simulink model "Practica_3_simulin_Simscape"  (R2022b)
settings: Solver=VariableStepAuto  StartTime=0.0  StopTime=10  FixedStep=0.001  MaxStep=0.00001  RelTol=1e-3
values from neighbouring files (symbols this model uses):
  b1 = 1000    [DobleP1.m]
  k1 = 16182    [DobleP1.m]
  k2 = 19000    [DobleP1.m]
  m1 = 290    [DobleP1.m]
  m2 = 59    [DobleP1.m]
libraries: fl_lib x11, nesl_utility x4
settings Model: Creator=mluser  LastModifiedBy=mluser

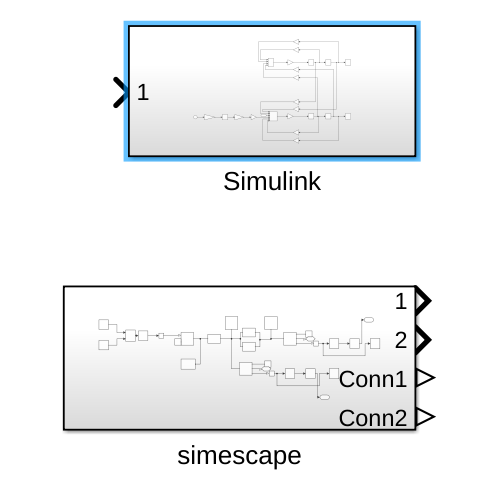
[thumbnail: Simulink's stored preview of the top-level diagram]
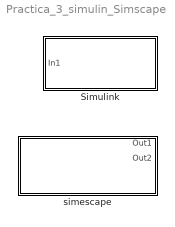
== system Practica_3_simulin_Simscape ==
  Simulink : Subsystem
  simescape : Subsystem

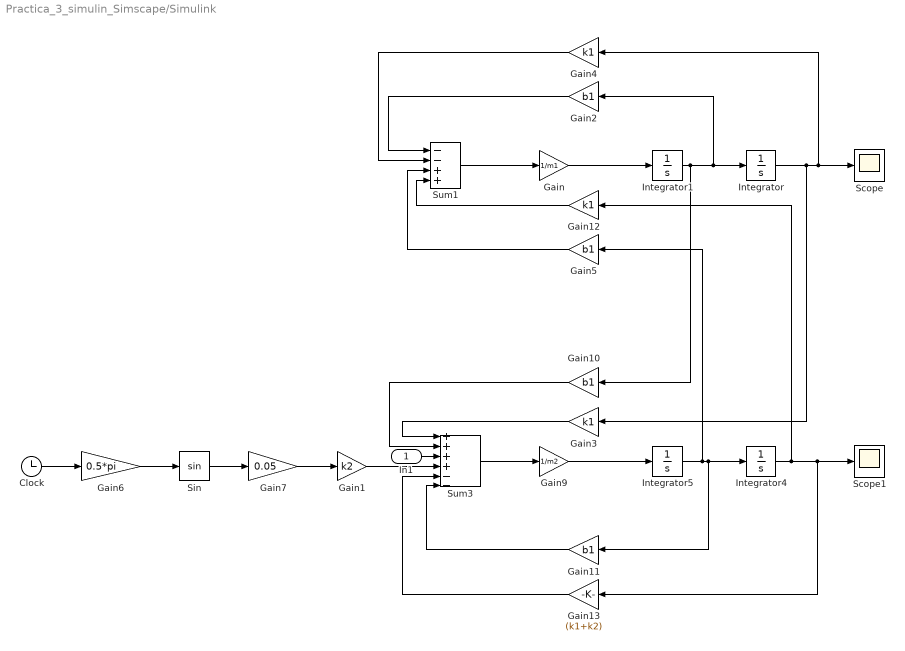
== system Practica_3_simulin_Simscape/Simulink ==
  In1 : Inport
  Clock : Clock
  Gain : Gain  Gain=1/m1
  Gain1 : Gain  Gain=k2
  Gain{2,5,10..11} (4 alike) : Gain  Gain=b1
  Gain12 : Gain  Gain=k1
  Gain13 : Gain  Gain=(k1+k2)
  Gain3 : Gain  Gain=k1
  Gain4 : Gain  Gain=k1
  Gain6 : Gain  Gain=0.5*pi
  Gain7 : Gain  Gain=0.05
  Gain9 : Gain  Gain=1/m2
  Integrator{,1,4..5} (4 alike) : Integrator
  Scope : Scope
  Scope1 : Scope
  Sin : Trigonometry
  Sum1 : Sum  Inputs=--++
  Sum3 : Sum  Inputs=++++--
  wires:
  Clock/1 -> Gain6/1
  Gain2/1 -> Sum1/1
  Sin/1 -> Gain7/1
  Gain9/1 -> Integrator5/1
  Gain10/1 -> Sum3/2
  Sum3/1 -> Gain9/1
  Gain/1 -> Integrator1/1
  Integrator/1 -> Gain4/1, Scope/1, Gain3/1
  Gain3/1 -> Sum3/1
  Gain5/1 -> Sum1/3
  Integrator4/1 -> Gain13/1, Scope1/1, Gain12/1
  Integrator5/1 -> Gain5/1, Gain11/1, Integrator4/1
  Gain11/1 -> Sum3/6
  Gain13/1 -> Sum3/5
  Gain1/1 -> Sum3/4
  Sum1/1 -> Gain/1
  Gain12/1 -> Sum1/4
  In1/1 -> Sum3/3
  Gain6/1 -> Sin/1
  Gain7/1 -> Gain1/1
  Integrator1/1 -> Gain2/1, Integrator/1, Gain10/1
  Gain4/1 -> Sum1/2

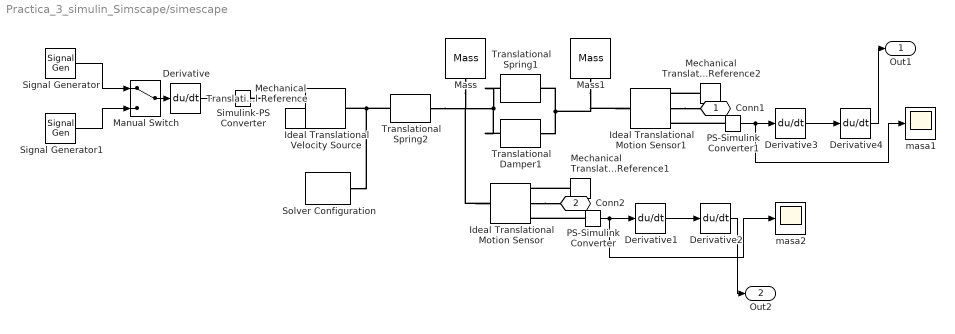
== system Practica_3_simulin_Simscape/simescape ==
  Derivative{,1..4} (5 alike) : Derivative
  Ideal Translational Motion Sensor : fl_lib/Mechanical/Mechanical Sensors/Ideal Translational Motion Sensor  reference=foundation.enum.MeasurementReference.difference  acceleration_port=false  velocity_port=true  position_port=true  offset=0 m
  Ideal Translational Motion Sensor1 : fl_lib/Mechanical/Mechanical Sensors/Ideal Translational Motion Sensor  reference=foundation.enum.MeasurementReference.difference  acceleration_port=false  velocity_port=true  position_port=true  offset=0 m
  Ideal Translational Velocity Source : fl_lib/Mechanical/Mechanical Sources/Ideal Translational Velocity Source
  Manual Switch : ManualSwitch
  Mass : fl_lib/Mechanical/Translational Elements/Mass  mass=59 kg  num_ports=foundation.enum.numPorts2.one  v_specify=off  v_priority=High  v=0 m/s  v_nominal_specify=off  v_nominal_unit=m/s  v_nominal_value=1  f_specify=off  f_priority=None  f=0 N  f_nominal_specify=off  f_nominal_unit=N  f_nominal_value=1
  Mass1 : fl_lib/Mechanical/Translational Elements/Mass  mass=290 kg  num_ports=foundation.enum.numPorts2.one  v_specify=off  v_priority=High  v=0 m/s  v_nominal_specify=off  v_nominal_unit=m/s  v_nominal_value=1  f_specify=off  f_priority=None  f=0 N  f_nominal_specify=off  f_nominal_unit=N  f_nominal_value=1
  Mechanical Translational Reference : fl_lib/Mechanical/Translational Elements/Mechanical Translational Reference
  Mechanical Translational Reference1 : fl_lib/Mechanical/Translational Elements/Mechanical Translational Reference
  Mechanical Translational Reference2 : fl_lib/Mechanical/Translational Elements/Mechanical Translational Reference
  PS-Simulink Converter : nesl_utility/PS-Simulink Converter  PhysicalDomain=network_engine_domain  SubClassName=ps_output  LeftPortType=input  RightPortType=output  PseudoPeriodic=off  Frequencies=[]  VectorFormat=inherit  Unit=inherit  AffineConversion=off
  PS-Simulink Converter1 : nesl_utility/PS-Simulink Converter  PhysicalDomain=network_engine_domain  SubClassName=ps_output  LeftPortType=input  RightPortType=output  PseudoPeriodic=off  Frequencies=[]  VectorFormat=inherit  Unit=inherit  AffineConversion=off
  Signal Generator : SignalGenerator  Amplitude=0.05  Frequency=0.5*pi  Units=rad/sec
  Signal Generator1 : SignalGenerator  Amplitude=0.05  Frequency=20*pi  Units=rad/sec
  Simulink-PS Converter : nesl_utility/Simulink-PS Converter  PhysicalDomain=network_engine_domain  SubClassName=ps_input  LeftPortType=input  RightPortType=output  PseudoPeriodic=off  Frequencies=[]  NoiseDistribution=none  NoiseParameters=[]  Unit=1  AffineConversion=off  FilteringAndDerivatives=provide  SimscapeFilterOrder=1  InputFilterTimeConstant=0.001  UdotUserProvided=0
  Solver Configuration : nesl_utility/Solver Configuration  PhysicalDomain=network_engine_domain  SubClassName=solver  LeftPortType=input  RightPortType=generic  Tones=[]  Harmonics=[]  SimulateNoise=off  Profile=off  UseLocalSampling=off  EnableSwitchedLinearOptims=on  FrequencyDomain=off  UseCCode=off  RelTol=0.001  AbsTol=0.001  MinStep=1e-09  ToWorkspace=off  RevertToSquareIcSolve=off  NumHomotopyIterations=100  PhasorMode=off  PhasorModeNumHarmonics=1  ConsistencySolver=NEWTON_XTOL_AFTER_FTOL  IndexReductionMethod=DerivativeReplacement  DoDC=off  ResidualTolerance=1e-09  ConsistencyTolSource=GLOBAL  ConsistencyAbsTol=0.001  ConsistencyRelTol=0.001  ConsistencyTolFactor=0.001  UseLocalSolver=off  LocalSolverChoice=NE_BACKWARD_EULER_ADVANCER  ResolveIndetEquations=on  FunctionEvalNumThread=1  LocalSolverSampleTime=0.001  DoFixedCost=off  MaxNonlinIter=3  MaxModeIter=2  ComputeImpulses=off  ImpulseIterations=2  LinearAlgebra=auto  LinearAlgebraNumThread=0  EquationFormulation=NE_TIME_EF  DelaysMemoryBudget=1024  AutomaticFiltering=on  FilteringTimeConstant=0.001  PartitionStorageMethod=AS_NEEDED  PartitionMemoryBudget=1024  PartitionMethod=ROBUST
  Translational Damper1 : fl_lib/Mechanical/Translational Elements/Translational Damper  D=1000 N*s/m  v_specify=off  v_priority=None  v=0 m/s  v_nominal_specify=off  v_nominal_unit=m/s  v_nominal_value=1  f_specify=off  f_priority=None  f=0 N  f_nominal_specify=off  f_nominal_unit=N  f_nominal_value=1
  Translational Spring1 : fl_lib/Mechanical/Translational Elements/Translational Spring  spr_rate=16182 N/m  v_specify=off  v_priority=None  v=0 m/s  v_nominal_specify=off  v_nominal_unit=m/s  v_nominal_value=1  f_specify=off  f_priority=None  f=0 N  f_nominal_specify=off  f_nominal_unit=N  f_nominal_value=1  x_specify=off  x_priority=High  x=0 m  x_nominal_specify=off  x_nominal_unit=m  x_nominal_value=1
  Translational Spring2 : fl_lib/Mechanical/Translational Elements/Translational Spring  spr_rate=19000 N/m  v_specify=off  v_priority=None  v=0 m/s  v_nominal_specify=off  v_nominal_unit=m/s  v_nominal_value=1  f_specify=off  f_priority=None  f=0 N  f_nominal_specify=off  f_nominal_unit=N  f_nominal_value=1  x_specify=off  x_priority=High  x=0 m  x_nominal_specify=off  x_nominal_unit=m  x_nominal_value=1
  masa1 : Scope
  masa2 : Scope
  Conn1 : PMIOPort  Side=Right
  Conn2 : PMIOPort  Port=2  Side=Right
  Out1 : Outport
  Out2 : Outport  Port=2
  wires:
  Derivative1/1 -> Derivative2/1
  Derivative3/1 -> Derivative4/1
  Derivative/1 -> Simulink-PS Converter/1
  Signal Generator1/1 -> Manual Switch/2
  Derivative4/1 -> Out1/1
  Derivative2/1 -> Out2/1
  Manual Switch/1 -> Derivative/1
  PS-Simulink Converter1/1 -> masa1/1, Derivative3/1
  PS-Simulink Converter/1 -> masa2/1, Derivative1/1
  Signal Generator/1 -> Manual Switch/1
  connections:
  Ideal Translational Velocity Source/RConn1 -- Simulink-PS Converter/RConn1
  Ideal Translational Motion Sensor/RConn2 -- Conn2/RConn1
  Ideal Translational Motion Sensor1/RConn2 -- Conn1/RConn1
  PS-Simulink Converter/LConn1 -- Ideal Translational Motion Sensor/RConn3
  Translational Damper1/RConn1 -- Ideal Translational Motion Sensor1/LConn1 -- Mass1/LConn1 -- Translational Spring1/RConn1
  Mechanical Translational Reference/LConn1 -- Ideal Translational Velocity Source/RConn2
  Mechanical Translational Reference2/LConn1 -- Ideal Translational Motion Sensor1/RConn1
  Translational Spring1/LConn1 -- Ideal Translational Motion Sensor/LConn1 -- Mass/LConn1 -- Translational Spring2/RConn1 -- Translational Damper1/LConn1
  PS-Simulink Converter1/LConn1 -- Ideal Translational Motion Sensor1/RConn3
  Mechanical Translational Reference1/LConn1 -- Ideal Translational Motion Sensor/RConn1
  Translational Spring2/LConn1 -- Solver Configuration/RConn1 -- Ideal Translational Velocity Source/LConn1
